simulink model "Filter_attivo"  (R2016b)
settings: Solver=ode23t  StartTime=0.0  StopTime=2.4  MaxStep=1e-4  RelTol=1e-3  EnableMultiTasking=on
values from neighbouring files (symbols this model uses):
  ampiezza_rete = 150/sqrt(3)    [Data.m]    (also in taratura.m)
  C = 2.2e-3    (= 0.0022)    [Data.m]
  C_raddr = 600e-6    (= 0.0006)    [Data.m]
  f = 50    [Data.m]    (also in Spettro_complesso.m = bar(-fp((26:25:25000-25)),PyTHD(length(PyTHD)-1:-1:length(Py)
  f_am = 500    [Data.m]
  h = Lagrange_coef(f,1/Tc)    [Data.m]    (also in Lagrange_coef.m = NaN(4,round(fc/f1*0.5)))
  h_rit = Lagrange_coef_rit(1.5)    [Data.m]
  k_interno = 0.99    [tuning.m]
  k_par_AM = 10    [Data.m]
  ki_PI = 0.2    [Data.m]
  ki_PLL = 1000    [Data.m]
  ki_ris = 47.5*2    (= 95)    [Data.m]
  kp_PI = 1.57    [Data.m]
  kp_PLL = 0.9    [Data.m]
  kp_ris = 47.5*0.089*2    (= 8.455)    [Data.m]
  L_disaccoppiamento = 2*1.18e-3    (= 0.00236)    [Data.m]    (also in taratura.m)
  L_rete = 4e-3    (= 0.004)    [Data.m]    (also in tuning.m)
  max_PI = 8    [Data.m]
  max_PLL = 1000    [Data.m]
  min_PI = -8    [Data.m]
  min_PLL = -1000    [Data.m]
  Notch_z = 1-Peaking_z    [Data.m]
  Notch_z_AM1 = 1-Peaking_z_AM1    [Notch.m]
  peak_rete = Peaking(f,1/Tc,0.1)    [Data.m]
  Peaking_dir1_d = c2d(Peaking_dir1_s,1/fs,'tustin')    [semipeaking.m]
  pendenza = 1000    [Data.m]
  R_carico = 50    [Data.m]
  R_disaccoppiamento = 2*13e-3    (= 0.026)    [Data.m]    (also in taratura.m)
  R_raddr = 60    [Data.m]
  R_rete = 100e-3    (= 0.1)    [Data.m]    (also in tuning.m = 0.01)
  T = 20e-3    (= 0.02)    [Data.m]    (also in tuning.m)
  tau_filtro_Vdc_ref = 0.15    [Data.m]
  Tc = 1/10000    (= 0.0001)    [Data.m]    (also in taratura.m; tuning.m)
  Vdc_ref = 200    [Data.m]    (also in taratura.m)
  w_filtro = 2*pi*f_taglio    (= 56548.6677646)    [Data.m]
undefined symbols (not defined in the file or in its folder): DiscIntNeverNeededParam, k_par, k_ser, Notch_z_AM1_5, Notch_z_AM1_7, Notch_z_AM2_5, Notch_z_AM2_7, Peaking_inv_d, plecs, Q_inv
libraries: powerlib x54, simulink x8, powerlib_extras x4, powerlib_meascontrol x2
(part 2 of 5)

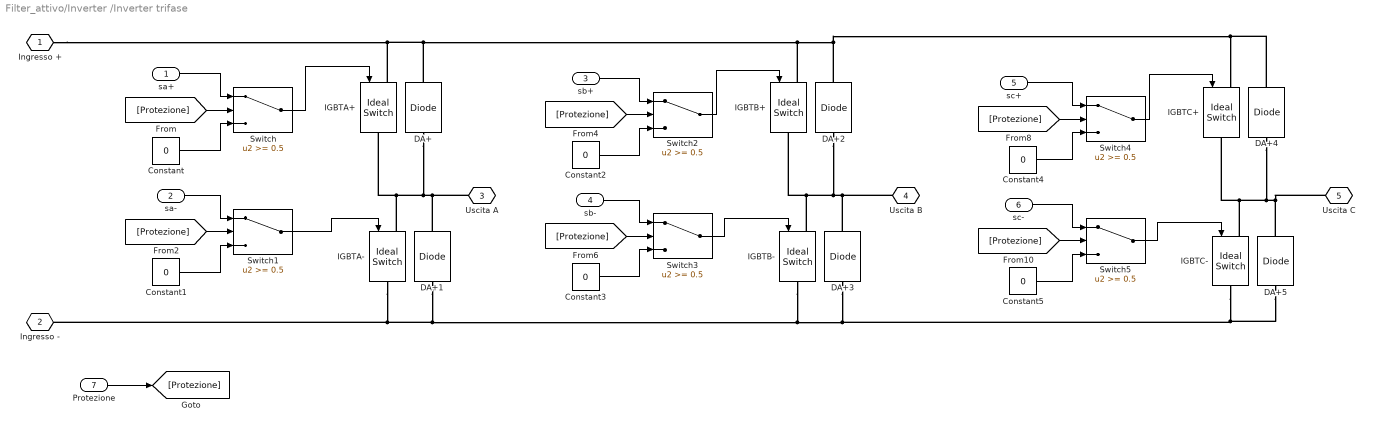
== system Filter_attivo/Inverter /Inverter trifase ==
  sa+ : Inport
  sa- : Inport  Port=2
  sb+ : Inport  Port=3
  sb- : Inport  Port=4
  sc+ : Inport  Port=5
  sc- : Inport  Port=6
  Protezione : Inport  Port=7
  Constant{,1..5} (6 alike) : Constant  Value=0
  DA+{,1..5} (6 alike) : powerlib/Power Electronics/Diode  Ron=Resistance_D  Lon=0  Vf=Forw_volt_d  IC=0  UseSnubber=off  Rs=500  Cs=250e-9  Measurements=off
  IGBTA+ : powerlib/Power Electronics/Ideal Switch  Ron=Int_res  Lon=0  IC=0  Rs=Snubber_res  Cs=inf  Measurements=off
  IGBTA- : powerlib/Power Electronics/Ideal Switch  Ron=Int_res  Lon=0  IC=0  Rs=Snubber_res  Cs=inf  Measurements=off
  IGBTB+ : powerlib/Power Electronics/Ideal Switch  Ron=Int_res  Lon=0  IC=0  Rs=Snubber_res  Cs=inf  Measurements=off
  IGBTB- : powerlib/Power Electronics/Ideal Switch  Ron=Int_res  Lon=0  IC=0  Rs=Snubber_res  Cs=inf  Measurements=off
  IGBTC+ : powerlib/Power Electronics/Ideal Switch  Ron=Int_res  Lon=0  IC=0  Rs=Snubber_res  Cs=inf  Measurements=off
  IGBTC- : powerlib/Power Electronics/Ideal Switch  Ron=Int_res  Lon=0  IC=0  Rs=Snubber_res  Cs=inf  Measurements=off
  Switch{,1..5} (6 alike) : Switch  Threshold=0.5
  Ingresso + : PMIOPort  Tag=PMCPort  Port=1  Side=Left
  Ingresso - : PMIOPort  Tag=PMCPort  Port=2  Side=Left
  Uscita A : PMIOPort  Tag=PMCPort  Port=3  Side=Right
  Uscita B : PMIOPort  Tag=PMCPort  Port=4  Side=Right
  Uscita C : PMIOPort  Tag=PMCPort  Port=5  Side=Right
  wires:
  Switch/1 -> IGBTA+/1
  [Protezione] -> Switch/2
  sa+/1 -> Switch/1
  sa-/1 -> Switch1/1
  [Protezione] -> Switch1/2
  [Protezione] -> Switch2/2
  sb+/1 -> Switch2/1
  sb-/1 -> Switch3/1
  [Protezione] -> Switch3/2
  [Protezione] -> Switch4/2
  sc+/1 -> Switch4/1
  sc-/1 -> Switch5/1
  [Protezione] -> Switch5/2
  Constant/1 -> Switch/3
  Constant1/1 -> Switch1/3
  Constant2/1 -> Switch2/3
  Constant3/1 -> Switch3/3
  Constant4/1 -> Switch4/3
  Constant5/1 -> Switch5/3
  Protezione/1 -> [Protezione]
  Switch1/1 -> IGBTA-/1
  Switch3/1 -> IGBTB-/1
  Switch2/1 -> IGBTB+/1
  Switch5/1 -> IGBTC-/1
  Switch4/1 -> IGBTC+/1
  connections:
  DA+1/LConn1 -- IGBTA-/RConn1 -- Ingresso -/RConn1 -- IGBTB-/RConn1 -- DA+5/LConn1 -- IGBTC-/RConn1 -- DA+3/LConn1
  DA+/LConn1 -- DA+1/RConn1 -- Uscita A/RConn1 -- IGBTA-/LConn1 -- IGBTA+/RConn1
  IGBTA+/LConn1 -- Ingresso +/RConn1 -- DA+/RConn1 -- IGBTB+/LConn1 -- DA+4/RConn1 -- IGBTC+/LConn1 -- DA+2/RConn1
  IGBTB+/RConn1 -- IGBTB-/LConn1 -- Uscita B/RConn1 -- DA+3/RConn1 -- DA+2/LConn1
  IGBTC+/RConn1 -- IGBTC-/LConn1 -- Uscita C/RConn1 -- DA+5/RConn1 -- DA+4/LConn1

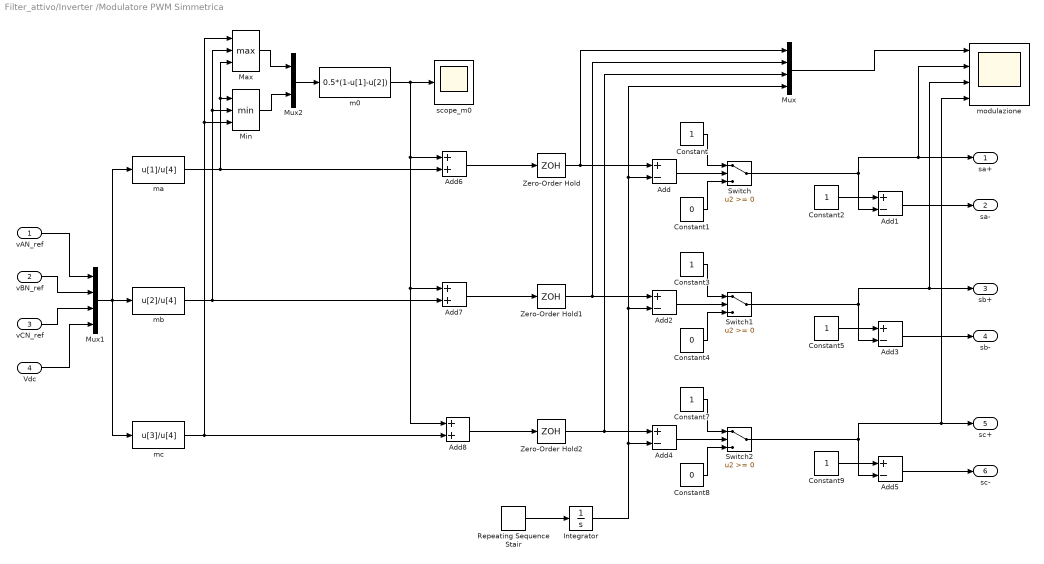
== system Filter_attivo/Inverter /Modulatore PWM Simmetrica ==
  vAN_ref : Inport
  vBN_ref : Inport  Port=2
  vCN_ref : Inport  Port=3
  Vdc : Inport  Port=4
  Add{,1..5} (6 alike) : Sum  Inputs=+-
  Add6 : Sum
  Add7 : Sum
  Add8 : Sum
  Constant{,2..3,5,7,9} (6 alike) : Constant
  Constant1 : Constant  Value=0
  Constant4 : Constant  Value=0
  Constant8 : Constant  Value=0
  Integrator : Integrator
  Max : MinMax  Function=max  Inputs=3
  Min : MinMax  Inputs=3
  Mux : Mux
  Mux1 : Mux
  Mux2 : Mux  Inputs=2
  Repeating Sequence Stair : simulink/Sources/Repeating Sequence Stair  OutValues=[2/Tc -2/Tc].'  tsamp=Tc/2  OutMin=[]  OutMax=[]  OutDataTypeStr=float('double')  OutputDataTypeScalingMode=Specify via dialog  OutDataType=float('double')  ConRadixGroup=Best Precision: Vector-wise  OutScaling=2^-12
  Switch : Switch
  Switch1 : Switch
  Switch2 : Switch
  Zero-Order Hold : ZeroOrderHold  SampleTime=Tc
  Zero-Order Hold1 : ZeroOrderHold  SampleTime=Tc
  Zero-Order Hold2 : ZeroOrderHold  SampleTime=Tc
  m0 : Fcn  Expr=0.5*(1-u[1]-u[2])
  ma : Fcn  Expr=u[1]/u[4]
  mb : Fcn  Expr=u[2]/u[4]
  mc : Fcn  Expr=u[3]/u[4]
  modulazione : Scope  NumInputPorts=4
  scope_m0 : Scope
  sa+ : Outport
  sa- : Outport  Port=2
  sb+ : Outport  Port=3
  sb- : Outport  Port=4
  sc+ : Outport  Port=5
  sc- : Outport  Port=6
  wires:
  Zero-Order Hold/1 -> Add/1, Mux/1
  Integrator/1 -> Add2/2, Add/2, Mux/4, Add4/2
  Add/1 -> Switch/2
  Constant/1 -> Switch/1
  Constant1/1 -> Switch/3
  Switch/1 -> Add1/2, sa+/1, modulazione/2
  Constant2/1 -> Add1/1
  Add1/1 -> sa-/1
  Repeating Sequence Stair/1 -> Integrator/1
  Zero-Order Hold1/1 -> Add2/1, Mux/2
  Add2/1 -> Switch1/2
  Constant3/1 -> Switch1/1
  Constant4/1 -> Switch1/3
  Switch1/1 -> Add3/2, sb+/1, modulazione/3
  Constant5/1 -> Add3/1
  Add3/1 -> sb-/1
  vAN_ref/1 -> Mux1/1
  vBN_ref/1 -> Mux1/2
  vCN_ref/1 -> Mux1/3
  Vdc/1 -> Mux1/4
  Zero-Order Hold2/1 -> Add4/1, Mux/3
  Add4/1 -> Switch2/2
  Constant7/1 -> Switch2/1
  Constant8/1 -> Switch2/3
  Switch2/1 -> Add5/2, sc+/1, modulazione/4
  Constant9/1 -> Add5/1
  Add5/1 -> sc-/1
  Mux1/1 -> ma/1, mc/1, mb/1
  Mux/1 -> modulazione/1
  mb/1 -> Min/2, Max/2, Add7/2
  mc/1 -> Min/3, Max/1, Add8/2
  ma/1 -> Min/1, Max/3, Add6/2
  Min/1 -> Mux2/2
  Max/1 -> Mux2/1
  Add6/1 -> Zero-Order Hold/1
  Add8/1 -> Zero-Order Hold2/1
  Add7/1 -> Zero-Order Hold1/1
  m0/1 -> scope_m0/1, Add6/1, Add7/1, Add8/1
  Mux2/1 -> m0/1

== system Filter_attivo/Inverter /Scope_idc ==
  1 : Inport
  " InputMux " : Subsystem
      mask Display: disp('Mux')
  " S-Function " : S-Function  FunctionName=plecs  SFunctionDeploymentMode=off  EnableBusSupport=off
  wires:
  " InputMux "/1(Out) -> " S-Function "/1
  1/1 -> " InputMux "/1(In1)

== system Filter_attivo/Inverter /Scope_idc_media ==
  1 : Inport
  " InputMux " : Subsystem
      mask Display: disp('Mux')
  " S-Function " : S-Function  FunctionName=plecs  SFunctionDeploymentMode=off  EnableBusSupport=off
  wires:
  1/1 -> " InputMux "/1(In1)
  " InputMux "/1(Out) -> " S-Function "/1

== system Filter_attivo/Protezione/Scope ==
  1 : Inport
  2 : Inport  Port=2
  3 : Inport  Port=3
  " 1 " : DataTypeConversion  SaturateOnIntegerOverflow=on  RndMeth=Zero
  " 2 " : DataTypeConversion  SaturateOnIntegerOverflow=on  RndMeth=Zero
  " 3 " : DataTypeConversion  SaturateOnIntegerOverflow=on  RndMeth=Zero
  " InputMux " : Mux  Inputs=3
  " S-Function " : S-Function  FunctionName=plecs  SFunctionDeploymentMode=off  EnableBusSupport=off
  wires:
  " InputMux "/1 -> " S-Function "/1
  1/1 -> " 1 "/1
  " 1 "/1 -> " InputMux "/1
  2/1 -> " 2 "/1
  " 2 "/1 -> " InputMux "/2
  3/1 -> " 3 "/1
  " 3 "/1 -> " InputMux "/3

== system Filter_attivo/Rete/D ==
  ab(c) : Inport
  Gain : Gain  Gain=[1 0; 1/sqrt(3) 2/sqrt(3)]  Multiplication=Matrix(K*u)
  dq(0) : Outport
  wires:
  Gain/1 -> dq(0)/1
  ab(c)/1 -> Gain/1

== system Filter_attivo/Rete/Integratore discreto con reset a 2*pi ==
  omega : Inport
  Add : Sum
  Compare To Zero : simulink/Logic and Bit Operations/Compare To Zero  relop=>  OutDataTypeStr=uint8  ZeroCross=off
  Constant : Constant  Value=2*pi
  Constant1 : Constant  Value=-2*pi
  Constant2 : Constant  Value=-2*pi
  Constant3 : Constant  Value=2*pi
  Discrete-Time Integrator : DiscreteIntegrator  ExternalReset=rising  InitialConditionSource=external  SampleTime=Tc  ShowStatePort=on  ICPrevOutput=DiscIntNeverNeededParam  ICPrevScaledInput=DiscIntNeverNeededParam
  Logical Operator2 : Logic  Operator=OR  AllPortsSameDT=off  OutDataTypeStr=boolean
  Relational Operator : RelationalOperator  Operator=<=  OutDataTypeStr=boolean  RndMeth=Nearest
  Relational Operator1 : RelationalOperator  Operator=<=  OutDataTypeStr=boolean  RndMeth=Nearest
  Switch : Switch  Threshold=0.5
  teta : Outport
  wires:
  Logical Operator2/1 -> Discrete-Time Integrator/2
  Relational Operator/1 -> Logical Operator2/1
  Relational Operator1/1 -> Logical Operator2/2
  Discrete-Time Integrator/State -> Add/1, Compare To Zero/1, Relational Operator1/1, Relational Operator/2
  Constant/1 -> Relational Operator/1
  Constant1/1 -> Relational Operator1/2
  omega/1 -> Discrete-Time Integrator/1
  Discrete-Time Integrator/1 -> teta/1
  Constant2/1 -> Switch/1
  Constant3/1 -> Switch/3
  Switch/1 -> Add/2
  Compare To Zero/1 -> Switch/2
  Add/1 -> Discrete-Time Integrator/3

== system Filter_attivo/Rete/generatore diretta e inversa ==
  note: c'è un disagio forte, perchè tutto il sistema è sincronizzato con una inversa e non con una diretta.
  Frequenza1 : Constant  Value=fase_i
  Frequenza2 : Constant  Value=f
  Gain1 : Gain  Gain=2*pi
  Gain2 : Gain  Gain=ampiezza_i
  Gain3 : Gain  Gain=pi/180
  MATLAB Function : MATLAB Function  TreatAsAtomicUnit=on
  Mux : Mux  Inputs=3
  Ramp2 : simulink/Sources/Ramp  slope=pendenza  start=0  X0=0
  Scope1 : Subsystem  LoadFcn=plecs('sl', 300);  InitFcn=plecs('sl', 314);  StartFcn=plecs('sl', 308);  StopFcn=plecs('sl', 309);  mask{Settings=<binary blob, 876 chars, not shown>}
      mask init:
      | plecs('sl', 315);
      settings: CopyFcn=plecs('sl', 303);  DeleteFcn=plecs('sl', 305);  UndoDeleteFcn=plecs('sl', 306);  PreSaveFcn=plecs('sl', 311);  NameChangeFcn=plecs('sl', 310);  DestroyFcn=plecs('sl', 307);  OpenFcn=plecs('sl', 302);  ErrorFcn=plerrorfcn
      mask Display: plot([0.1 0.9 0.9 0.1 0.1], [0.9 0.9 0.5 0.5 0.9])
  Step3 : Step  Time=0  After=ampiezza_rete  SampleTime=0
  Switch3 : Switch  Threshold=ampiezza_rete
  "integratore con reset " : Subsystem
  v_a : Outport
  v_b : Outport  Port=2
  v_c : Outport  Port=3
  wires:
  Gain1/1 -> "integratore con reset "/1(omega)
  Ramp2/1 -> Switch3/2, Switch3/3
  Step3/1 -> Switch3/1
  Frequenza2/1 -> Gain1/1
  "integratore con reset "/1(teta) -> MATLAB Function/1(teta)
  Switch3/1 -> Gain2/1, MATLAB Function/2(a_d)
  MATLAB Function/1(v_a) -> Mux/1, v_a/1
  MATLAB Function/3(v_c) -> Mux/3, v_b/1
  MATLAB Function/2(v_b) -> Mux/2, v_c/1
  Gain2/1 -> MATLAB Function/3(a_i)
  Frequenza1/1 -> Gain3/1
  Mux/1 -> Scope1/1(1)
  Gain3/1 -> MATLAB Function/4(fase_i)

== system Filter_attivo/Scope1/ InputMux  ==
  In1 : Inport
  Convert1 : DataTypeConversion  SaturateOnIntegerOverflow=on  RndMeth=Zero
  Mux : Mux  Inputs=1
  Out : Outport
  wires:
  Convert1/1 -> Mux/1
  In1/1 -> Convert1/1
  Mux/1 -> Out/1

== system Filter_attivo/Scope2/ InputMux  ==
  In1 : Inport
  Convert1 : DataTypeConversion  SaturateOnIntegerOverflow=on  RndMeth=Zero
  Mux : Mux  Inputs=1
  Out : Outport
  wires:
  Mux/1 -> Out/1
  In1/1 -> Convert1/1
  Convert1/1 -> Mux/1

== system Filter_attivo/Tensione bus DC/ InputMux  ==
  In1 : Inport
  Convert1 : DataTypeConversion  SaturateOnIntegerOverflow=on  RndMeth=Zero
  Mux : Mux  Inputs=1
  Out : Outport
  wires:
  Convert1/1 -> Mux/1
  In1/1 -> Convert1/1
  Mux/1 -> Out/1

== system Filter_attivo/XY Plot/ InputMux  ==
  In1 : Inport
  In2 : Inport  Port=2
  Convert1 : DataTypeConversion  SaturateOnIntegerOverflow=on  RndMeth=Zero
  Convert2 : DataTypeConversion  SaturateOnIntegerOverflow=on  RndMeth=Zero
  Mux : Mux  Inputs=2
  Out : Outport
  wires:
  Convert2/1 -> Mux/2
  In2/1 -> Convert2/1
  Convert1/1 -> Mux/1
  In1/1 -> Convert1/1
  Mux/1 -> Out/1

== system Filter_attivo/v_rete/ InputMux  ==
  In1 : Inport
  Convert1 : DataTypeConversion  SaturateOnIntegerOverflow=on  RndMeth=Zero
  Mux : Mux  Inputs=1
  Out : Outport
  wires:
  Mux/1 -> Out/1
  In1/1 -> Convert1/1
  Convert1/1 -> Mux/1

== system Filter_attivo/v_rete1/ InputMux  ==
  In1 : Inport
  Convert1 : DataTypeConversion  SaturateOnIntegerOverflow=on  RndMeth=Zero
  Mux : Mux  Inputs=1
  Out : Outport
  wires:
  Convert1/1 -> Mux/1
  In1/1 -> Convert1/1
  Mux/1 -> Out/1

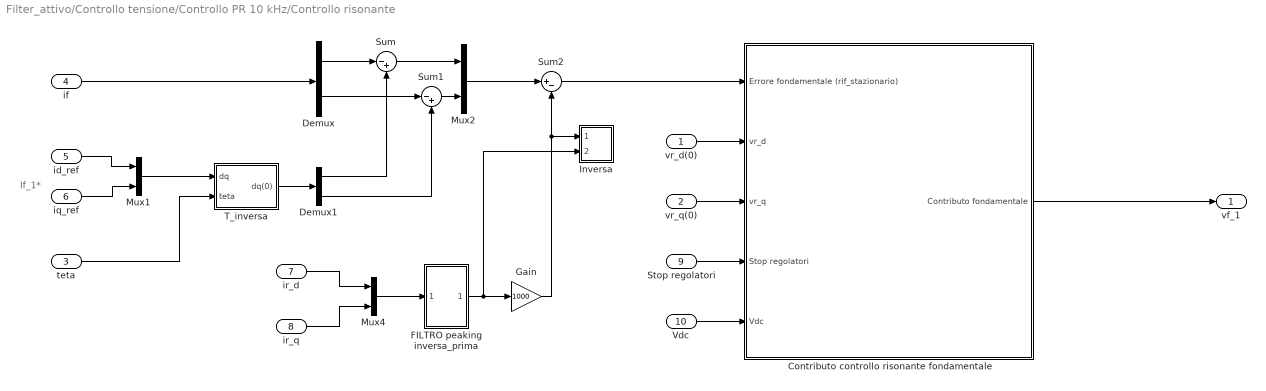
== system Filter_attivo/Controllo tensione/Controllo PR 10 kHz/Controllo risonante ==
  note: If_1*
  vr_d(0) : Inport
  vr_q(0) : Inport  Port=2
  teta : Inport  Port=3
  if : Inport  Port=4
  id_ref : Inport  Port=5
  iq_ref : Inport  Port=6
  ir_d : Inport  Port=7
  ir_q : Inport  Port=8
  Stop regolatori : Inport  Port=9
  Vdc : Inport  Port=10
  Contributo controllo risonante fondamentale : Subsystem
  Demux : Demux  Outputs=2
  Demux1 : Demux  Outputs=2
  FILTRO peaking inversa_prima : Subsystem
  Gain : Gain  Gain=1000
  Inversa : Subsystem  LoadFcn=plecs('sl', 300);  InitFcn=plecs('sl', 314);  StartFcn=plecs('sl', 308);  StopFcn=plecs('sl', 309);  mask{Settings=<binary blob, 1020 chars, not shown>}
      mask init:
      | plecs('sl', 315);
      settings: CopyFcn=plecs('sl', 303);  DeleteFcn=plecs('sl', 305);  UndoDeleteFcn=plecs('sl', 306);  PreSaveFcn=plecs('sl', 311);  NameChangeFcn=plecs('sl', 310);  DestroyFcn=plecs('sl', 307);  OpenFcn=plecs('sl', 302);  ErrorFcn=plerrorfcn
      mask Display: plot([0.1 0.9 0.9 0.1 0.1], [0.9 0.9 0.5 0.5 0.9])
  Mux1 : Mux  Inputs=2
  Mux2 : Mux  Inputs=2
  Mux4 : Mux  Inputs=2
  Sum : Sum  Inputs=|-+
  Sum1 : Sum  Inputs=|-+
  Sum2 : Sum  Inputs=|+-
  T_inversa : Subsystem
  vf_1 : Outport
  wires:
  Demux/1 -> Sum/1
  Demux/2 -> Sum1/1
  id_ref/1 -> Mux1/1
  iq_ref/1 -> Mux1/2
  Demux1/1 -> Sum/2
  Demux1/2 -> Sum1/2
  Sum/1 -> Mux2/1
  Sum1/1 -> Mux2/2
  vr_d(0)/1 -> Contributo controllo risonante fondamentale/2(vr_d)
  vr_q(0)/1 -> Contributo controllo risonante fondamentale/3(vr_q)
  Contributo controllo risonante fondamentale/1("Contributo fondamentale ") -> vf_1/1
  Mux2/1 -> Sum2/1
  teta/1 -> T_inversa/2(teta)
  Mux1/1 -> T_inversa/1(dq)
  T_inversa/1(dq(0)) -> Demux1/1
  Stop regolatori/1 -> Contributo controllo risonante fondamentale/4(Stop regolatori)
  Mux4/1 -> FILTRO peaking inversa_prima/1(In2)
  ir_d/1 -> Mux4/1
  ir_q/1 -> Mux4/2
  FILTRO peaking inversa_prima/1(Out1) -> Gain/1, Inversa/2(2)
  Gain/1 -> Sum2/2, Inversa/1(1)
  Sum2/1 -> Contributo controllo risonante fondamentale/1(Errore fondamentale (rif_stazionario))
  Vdc/1 -> Contributo controllo risonante fondamentale/5(Vdc)
  if/1 -> Demux/1

== system Filter_attivo/Controllo tensione/Controllo PR 10 kHz/D ==
  ab(c) : Inport
  Gain : Gain  Gain=[1 0; 1/sqrt(3) 2/sqrt(3)]  Multiplication=Matrix(K*u)
  dq(0) : Outport
  wires:
  Gain/1 -> dq(0)/1
  ab(c)/1 -> Gain/1

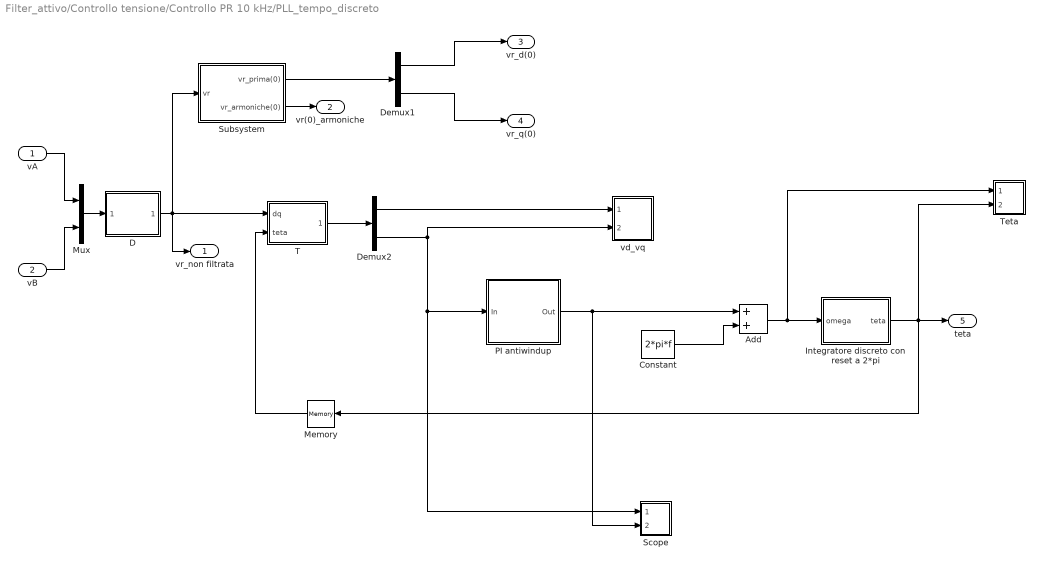
== system Filter_attivo/Controllo tensione/Controllo PR 10 kHz/PLL_tempo_discreto ==
  vA : Inport
  vB : Inport  Port=2
  Add : Sum
  Constant : Constant  Value=2*pi*f
  D : Subsystem
  Demux1 : Demux  Outputs=2
  Demux2 : Demux  Outputs=2
  Integratore discreto con reset a 2*pi : Subsystem
  Memory : Memory  InheritSampleTime=on
  Mux : Mux  Inputs=2
  PI antiwindup : Subsystem  mask{kp_PLL_edit=0.5, ki_PLL_edit=500}
      mask prompts: kp_PLL_edit "kp"; ki_PLL_edit "ki"
  Scope : Subsystem  LoadFcn=plecs('sl', 300);  InitFcn=plecs('sl', 314);  StartFcn=plecs('sl', 308);  StopFcn=plecs('sl', 309);  mask{Settings=<binary blob, 1004 chars, not shown>}
      mask init:
      | plecs('sl', 315);
      settings: CopyFcn=plecs('sl', 303);  DeleteFcn=plecs('sl', 305);  UndoDeleteFcn=plecs('sl', 306);  PreSaveFcn=plecs('sl', 311);  NameChangeFcn=plecs('sl', 310);  DestroyFcn=plecs('sl', 307);  OpenFcn=plecs('sl', 302);  ErrorFcn=plerrorfcn
      mask Display: plot([0.1 0.9 0.9 0.1 0.1], [0.9 0.9 0.5 0.5 0.9])
  Subsystem : Subsystem
  T : Subsystem
  Teta : Subsystem  LoadFcn=plecs('sl', 300);  InitFcn=plecs('sl', 314);  StartFcn=plecs('sl', 308);  StopFcn=plecs('sl', 309);  mask{Settings=<binary blob, 1020 chars, not shown>}
      mask init:
      | plecs('sl', 315);
      settings: CopyFcn=plecs('sl', 303);  DeleteFcn=plecs('sl', 305);  UndoDeleteFcn=plecs('sl', 306);  PreSaveFcn=plecs('sl', 311);  NameChangeFcn=plecs('sl', 310);  DestroyFcn=plecs('sl', 307);  OpenFcn=plecs('sl', 302);  ErrorFcn=plerrorfcn
      mask Display: plot([0.1 0.9 0.9 0.1 0.1], [0.9 0.9 0.5 0.5 0.9])
  vd_vq : Subsystem  LoadFcn=plecs('sl', 300);  InitFcn=plecs('sl', 314);  StartFcn=plecs('sl', 308);  StopFcn=plecs('sl', 309);  mask{Settings=<binary blob, 300 chars, not shown>}
      mask init:
      | plecs('sl', 315);
      settings: CopyFcn=plecs('sl', 303);  DeleteFcn=plecs('sl', 305);  UndoDeleteFcn=plecs('sl', 306);  PreSaveFcn=plecs('sl', 311);  NameChangeFcn=plecs('sl', 310);  DestroyFcn=plecs('sl', 307);  OpenFcn=plecs('sl', 302);  ErrorFcn=plerrorfcn
      mask Display: plot([0.1 0.9 0.9 0.1 0.1], [0.9 0.9 0.5 0.5 0.9])
  vr_non filtrata : Outport
  vr(0)_armoniche : Outport  Port=2
  vr_d(0) : Outport  Port=3
  vr_q(0) : Outport  Port=4
  teta : Outport  Port=5
  wires:
  Add/1 -> Teta/1(1), Integratore discreto con reset a 2*pi/1(omega)
  Constant/1 -> Add/2
  T/1(dq(teta)) -> Demux2/1
  Demux2/1 -> vd_vq/1(1)
  Integratore discreto con reset a 2*pi/1(teta) -> Memory/1, teta/1, Teta/2(2)
  Memory/1 -> T/2(teta)
  PI antiwindup/1(Out) -> Scope/2(2), Add/1
  vA/1 -> Mux/1
  vB/1 -> Mux/2
  Mux/1 -> D/1(ab(c))
  D/1(dq(0)) -> vr_non filtrata/1, Subsystem/1(vr), T/1(dq)
  Subsystem/2(vr_armoniche(0)) -> vr(0)_armoniche/1
  Demux1/1 -> vr_d(0)/1
  Demux1/2 -> vr_q(0)/1
  Subsystem/1(vr_prima(0)) -> Demux1/1
  Demux2/2 -> vd_vq/2(2), PI antiwindup/1(In), Scope/1(1)

== system Filter_attivo/Controllo tensione/Controllo PR 10 kHz/Scope ==
  1 : Inport
  " InputMux " : Subsystem
      mask Display: disp('Mux')
  " S-Function " : S-Function  FunctionName=plecs  SFunctionDeploymentMode=off  EnableBusSupport=off
  wires:
  1/1 -> " InputMux "/1(In1)
  " InputMux "/1(Out) -> " S-Function "/1

== system Filter_attivo/Controllo tensione/Controllo PR 10 kHz/Scope2 ==
  1 : Inport
  2 : Inport  Port=2
  " 1 " : DataTypeConversion  SaturateOnIntegerOverflow=on  RndMeth=Zero
  " 2 " : DataTypeConversion  SaturateOnIntegerOverflow=on  RndMeth=Zero
  " InputMux " : Mux  Inputs=2
  " S-Function " : S-Function  FunctionName=plecs  SFunctionDeploymentMode=off  EnableBusSupport=off
  wires:
  " InputMux "/1 -> " S-Function "/1
  1/1 -> " 1 "/1
  " 1 "/1 -> " InputMux "/1
  2/1 -> " 2 "/1
  " 2 "/1 -> " InputMux "/2

== system Filter_attivo/Controllo tensione/Controllo PR 10 kHz/controllo  ==
  teta : Inport
  ir : Inport  Port=2
  Demux : Demux  Outputs=2
  Mux : Mux  Inputs=2
  PI antiwindup : Subsystem  mask{kp_rifasamento=0.05, ki_rifasamento=5}
      mask prompts: kp_rifasamento "kp"; ki_rifasamento "ki"
  Peaking 1^ armonica : DiscreteTransferFcn  Numerator=cell2mat(peak_rete.num)  Denominator=cell2mat(peak_rete.den)
  Scope : Subsystem  LoadFcn=plecs('sl', 300);  InitFcn=plecs('sl', 314);  StartFcn=plecs('sl', 308);  StopFcn=plecs('sl', 309);  mask{Settings=<binary blob, 892 chars, not shown>}
      mask init:
      | plecs('sl', 315);
      settings: CopyFcn=plecs('sl', 303);  DeleteFcn=plecs('sl', 305);  UndoDeleteFcn=plecs('sl', 306);  PreSaveFcn=plecs('sl', 311);  NameChangeFcn=plecs('sl', 310);  DestroyFcn=plecs('sl', 307);  OpenFcn=plecs('sl', 302);  ErrorFcn=plerrorfcn
      mask Display: plot([0.1 0.9 0.9 0.1 0.1], [0.9 0.9 0.5 0.5 0.9])
  Scope1 : Subsystem  LoadFcn=plecs('sl', 300);  InitFcn=plecs('sl', 314);  StartFcn=plecs('sl', 308);  StopFcn=plecs('sl', 309);  mask{Settings=<binary blob, 892 chars, not shown>}
      mask init:
      | plecs('sl', 315);
      settings: CopyFcn=plecs('sl', 303);  DeleteFcn=plecs('sl', 305);  UndoDeleteFcn=plecs('sl', 306);  PreSaveFcn=plecs('sl', 311);  NameChangeFcn=plecs('sl', 310);  DestroyFcn=plecs('sl', 307);  OpenFcn=plecs('sl', 302);  ErrorFcn=plerrorfcn
      mask Display: plot([0.1 0.9 0.9 0.1 0.1], [0.9 0.9 0.5 0.5 0.9])
  Scope2 : Subsystem  LoadFcn=plecs('sl', 300);  InitFcn=plecs('sl', 314);  StartFcn=plecs('sl', 308);  StopFcn=plecs('sl', 309);  mask{Settings=<binary blob, 892 chars, not shown>}
      mask init:
      | plecs('sl', 315);
      settings: CopyFcn=plecs('sl', 303);  DeleteFcn=plecs('sl', 305);  UndoDeleteFcn=plecs('sl', 306);  PreSaveFcn=plecs('sl', 311);  NameChangeFcn=plecs('sl', 310);  DestroyFcn=plecs('sl', 307);  OpenFcn=plecs('sl', 302);  ErrorFcn=plerrorfcn
      mask Display: plot([0.1 0.9 0.9 0.1 0.1], [0.9 0.9 0.5 0.5 0.9])
  Scope3 : Subsystem  LoadFcn=plecs('sl', 300);  InitFcn=plecs('sl', 314);  StartFcn=plecs('sl', 308);  StopFcn=plecs('sl', 309);  mask{Settings=<binary blob, 892 chars, not shown>}
      mask init:
      | plecs('sl', 315);
      settings: CopyFcn=plecs('sl', 303);  DeleteFcn=plecs('sl', 305);  UndoDeleteFcn=plecs('sl', 306);  PreSaveFcn=plecs('sl', 311);  NameChangeFcn=plecs('sl', 310);  DestroyFcn=plecs('sl', 307);  OpenFcn=plecs('sl', 302);  ErrorFcn=plerrorfcn
      mask Display: plot([0.1 0.9 0.9 0.1 0.1], [0.9 0.9 0.5 0.5 0.9])
  Scope6 : Scope
  Step1 : Step  Time=avvio_rifasamento
  Sum5 : Sum  Inputs=|-+
  Switch : Switch  Criteria=u2 > Threshold
  T : Subsystem
  ir_q : Constant  Value=0
  ir_q1 : Constant  Value=0
  if_q* : Outport
  wires:
  Mux/1 -> Scope/1(1)
  ir/1 -> Peaking 1^ armonica/1
  T/1(dq(teta)) -> Scope1/1(1), Demux/1
  Sum5/1 -> PI antiwindup/1(In)
  Peaking 1^ armonica/1 -> Scope2/1(1), T/1(dq)
  Demux/2 -> Mux/2, Switch/1
  teta/1 -> T/2(teta)
  PI antiwindup/1(Out) -> Scope6/1, Scope3/1(1), if_q*/1
  ir_q/1 -> Mux/1, Sum5/2
  Switch/1 -> Sum5/1
  Step1/1 -> Switch/2
  ir_q1/1 -> Switch/3

== system Filter_attivo/Controllo tensione/Controllo PR 10 kHz/controllo bus DC ==
  Vdc : Inport
  Avvio Inverter : Inport  Port=2
  Filtro passa-basso tempo discreto : Subsystem
  PI antiwindup : Subsystem
  PI antiwindup1 : Subsystem  mask{kp_rifasamento=0.3, ki_rifasamento=0.01}
      mask prompts: kp_rifasamento "kp"; ki_rifasamento "ki"
  Scope1 : Subsystem  LoadFcn=plecs('sl', 300);  InitFcn=plecs('sl', 314);  StartFcn=plecs('sl', 308);  StopFcn=plecs('sl', 309);  mask{Settings=<binary blob, 904 chars, not shown>}
      mask init:
      | plecs('sl', 315);
      settings: CopyFcn=plecs('sl', 303);  DeleteFcn=plecs('sl', 305);  UndoDeleteFcn=plecs('sl', 306);  PreSaveFcn=plecs('sl', 311);  NameChangeFcn=plecs('sl', 310);  DestroyFcn=plecs('sl', 307);  OpenFcn=plecs('sl', 302);  ErrorFcn=plerrorfcn
      mask Display: plot([0.1 0.9 0.9 0.1 0.1], [0.9 0.9 0.5 0.5 0.9])
  Scope2 : Subsystem  LoadFcn=plecs('sl', 300);  InitFcn=plecs('sl', 314);  StartFcn=plecs('sl', 308);  StopFcn=plecs('sl', 309);  mask{Settings=<binary blob, 1076 chars, not shown>}
      mask init:
      | plecs('sl', 315);
      settings: CopyFcn=plecs('sl', 303);  DeleteFcn=plecs('sl', 305);  UndoDeleteFcn=plecs('sl', 306);  PreSaveFcn=plecs('sl', 311);  NameChangeFcn=plecs('sl', 310);  DestroyFcn=plecs('sl', 307);  OpenFcn=plecs('sl', 302);  ErrorFcn=plerrorfcn
      mask Display: plot([0.1 0.9 0.9 0.1 0.1], [0.9 0.9 0.5 0.5 0.9])
  Scope6 : Scope
  Sum5 : Sum  Inputs=|+-
  Vdc_ref : Constant  Value=Vdc_ref
  id* : Outport
  wires:
  Filtro passa-basso tempo discreto/1(Vdc*_filtrata) -> Scope2/1(1), Sum5/1
  Vdc_ref/1 -> Filtro passa-basso tempo discreto/1(In)
  Sum5/1 -> PI antiwindup1/1(In)
  Vdc/1 -> Filtro passa-basso tempo discreto/3("Vdc "), Sum5/2
  Avvio Inverter/1 -> Filtro passa-basso tempo discreto/2(Avvio Inverter)
  PI antiwindup1/1(Out) -> Scope1/1(1), Scope6/1, id*/1

== system Filter_attivo/Controllo tensione/Controllo ripetitivo/Controllo ripetitivo ==
  Stop regolatori : Inport
  Avvio ripetitivo : Inport  Port=2
  "corrente rete " : Inport  Port=3
  teta : Inport  Port=4
  Trigger : TriggerPort  VariantControl=Variant
  Demux : Demux  Outputs=2
  Logical Operator1 : Logic  AllPortsSameDT=off  OutDataTypeStr=boolean
  Mux2 : Mux  Inputs=2
  Regolatore ripetitivo : Subsystem
  vf_h : Outport
  wires:
  Mux2/1 -> vf_h/1
  Demux/1 -> Regolatore ripetitivo/1(id*)
  Demux/2 -> Regolatore ripetitivo/2(iq*)
  "corrente rete "/1 -> Demux/1
  Regolatore ripetitivo/2(Out2) -> Mux2/2
  Regolatore ripetitivo/1(Out1) -> Mux2/1
  Avvio ripetitivo/1 -> Logical Operator1/1
  Logical Operator1/1 -> Regolatore ripetitivo/Enable
  Stop regolatori/1 -> Logical Operator1/2
  teta/1 -> Regolatore ripetitivo/3(teta)

== system Filter_attivo/Controllo tensione/Controllo ripetitivo/Controllo ripetitivo con downsampling ==
  Stop regolatori : Inport
  Avvio ripetitivo : Inport  Port=2
  "corrente rete " : Inport  Port=3
  Trigger : TriggerPort  VariantControl=Variant
  And : Logic  AllPortsSameDT=off  OutDataTypeStr=boolean
  Demux : Demux  Outputs=2
  Mux2 : Mux  Inputs=2
  Regolatore ripetitivo : Subsystem
  vf_h_DOWNSAMPLING : Outport
  wires:
  Stop regolatori/1 -> And/2
  And/1 -> Regolatore ripetitivo/Enable
  Avvio ripetitivo/1 -> And/1
  Regolatore ripetitivo/1(Out1) -> Mux2/1
  Regolatore ripetitivo/2(Out2) -> Mux2/2
  "corrente rete "/1 -> Demux/1
  Demux/2 -> Regolatore ripetitivo/2(iq*)
  Demux/1 -> Regolatore ripetitivo/1(id*)
  Mux2/1 -> vf_h_DOWNSAMPLING/1

== system Filter_attivo/Controllo tensione/Controllo ripetitivo/Notch Prima Armonica ==
  ir(a_b_c) : Inport
  Trigger : TriggerPort  VariantControl=Variant
  D : Subsystem
  Demux : Demux  Outputs=2
  "Filtro notch prima armonica " : Subsystem
  Filtro notch prima armonica 1 : Subsystem
  Gain : Gain  Gain=0.1
  Gain1 : Gain  Gain=0.9
  Mux : Mux  Inputs=2
  Sum : Sum  Inputs=|++
  ir_h(d_q) : Outport
  wires:
  Demux/2 -> Filtro notch prima armonica 1/1(ir)
  Demux/1 -> "Filtro notch prima armonica "/1(ir)
  D/1(dq(0)) -> Gain/1, Demux/1
  ir(a_b_c)/1 -> D/1(ab(c))
  "Filtro notch prima armonica "/1(irh) -> Mux/1
  Filtro notch prima armonica 1/1(irh) -> Mux/2
  Mux/1 -> Gain1/1
  Sum/1 -> ir_h(d_q)/1
  Gain/1 -> Sum/2
  Gain1/1 -> Sum/1

== system Filter_attivo/Controllo tensione/Scope/ InputMux  ==
  In1 : Inport
  Convert1 : DataTypeConversion  SaturateOnIntegerOverflow=on  RndMeth=Zero
  Mux : Mux  Inputs=1
  Out : Outport
  wires:
  Convert1/1 -> Mux/1
  In1/1 -> Convert1/1
  Mux/1 -> Out/1

== system Filter_attivo/Controllo tensione/Scope2/ InputMux  ==
  In1 : Inport
  Convert1 : DataTypeConversion  SaturateOnIntegerOverflow=on  RndMeth=Zero
  Mux : Mux  Inputs=1
  Out : Outport
  wires:
  Convert1/1 -> Mux/1
  In1/1 -> Convert1/1
  Mux/1 -> Out/1

== system Filter_attivo/Inverter /Scope_idc/ InputMux  ==
  In1 : Inport
  Convert1 : DataTypeConversion  SaturateOnIntegerOverflow=on  RndMeth=Zero
  Mux : Mux  Inputs=1
  Out : Outport
  wires:
  Mux/1 -> Out/1
  In1/1 -> Convert1/1
  Convert1/1 -> Mux/1

== system Filter_attivo/Inverter /Scope_idc_media/ InputMux  ==
  In1 : Inport
  Convert1 : DataTypeConversion  SaturateOnIntegerOverflow=on  RndMeth=Zero
  Mux : Mux  Inputs=1
  Out : Outport
  wires:
  Convert1/1 -> Mux/1
  In1/1 -> Convert1/1
  Mux/1 -> Out/1

== system Filter_attivo/Rete/generatore diretta e inversa/Scope1 ==
  1 : Inport
  " InputMux " : Subsystem
      mask Display: disp('Mux')
  " S-Function " : S-Function  FunctionName=plecs  SFunctionDeploymentMode=off  EnableBusSupport=off
  wires:
  " InputMux "/1(Out) -> " S-Function "/1
  1/1 -> " InputMux "/1(In1)

== system Filter_attivo/Rete/generatore diretta e inversa/integratore con reset  ==
  omega : Inport
  Add : Sum
  Compare To Zero : simulink/Logic and Bit Operations/Compare To Zero  relop=>  OutDataTypeStr=uint8  ZeroCross=off
  Constant : Constant  Value=2*pi
  Constant1 : Constant  Value=-2*pi
  Constant2 : Constant  Value=-2*pi
  Constant3 : Constant  Value=2*pi
  Integrator : Integrator  ExternalReset=rising  InitialConditionSource=external  ShowStatePort=on
  Logical Operator2 : Logic  Operator=OR  AllPortsSameDT=off  OutDataTypeStr=boolean
  Relational Operator : RelationalOperator  Operator=<=  OutDataTypeStr=boolean  RndMeth=Nearest
  Relational Operator1 : RelationalOperator  Operator=<=  OutDataTypeStr=boolean  RndMeth=Nearest
  Switch : Switch  Threshold=0.5
  teta : Outport
  wires:
  Logical Operator2/1 -> Integrator/2
  Relational Operator/1 -> Logical Operator2/1
  Relational Operator1/1 -> Logical Operator2/2
  Integrator/State -> Add/1, Compare To Zero/1, Relational Operator1/1, Relational Operator/2
  Constant/1 -> Relational Operator/1
  Constant1/1 -> Relational Operator1/2
  omega/1 -> Integrator/1
  Integrator/1 -> teta/1
  Constant2/1 -> Switch/1
  Constant3/1 -> Switch/3
  Switch/1 -> Add/2
  Compare To Zero/1 -> Switch/2
  Add/1 -> Integrator/3

== system Filter_attivo/Controllo tensione/Controllo PR 10 kHz/Controllo risonante/Contributo controllo risonante fondamentale ==
  note: vf1_q*
  note: vf1_d*
  Errore fondamentale (rif_stazionario) : Inport
  vr_d : Inport  Port=2
  vr_q : Inport  Port=3
  Stop regolatori : Inport  Port=4
  Vdc : Inport  Port=5
  Add : Sum  Inputs=-+
  Add1 : Sum  Inputs=+-
  Demux1 : Demux  Outputs=2
  Demux3 : Demux  Outputs=2
  Logical Operator : Logic  Operator=NOT  AllPortsSameDT=off  OutDataTypeStr=boolean
  Mux1 : Mux  Inputs=2
  Mux2 : Mux  Inputs=2
  PIR_tustin_prewarp : Subsystem  Commented=on  mask{w_ris=2*pi*f, kr_ris=ki_ris, kp_ris=kp_ris, Tc=Tc, delta=0}
      mask prompts: w_ris "frequenza risonanza"; kr_ris "guadagno risonante"; kp_ris "guadagno proporzionale"; Tc "Periodo di campionamento"; delta "attenuazione"
  PI_risonante : Subsystem
  "Contributo fondamentale " : Outport
  wires:
  Errore fondamentale (rif_stazionario)/1 -> Demux1/1
  Stop regolatori/1 -> Logical Operator/1
  vr_d/1 -> Add/2
  Demux3/2 -> Add1/2
  vr_q/1 -> Add1/1
  Mux2/1 -> Demux3/1
  Mux1/1 -> "Contributo fondamentale "/1
  Demux3/1 -> Add/1
  Vdc/1 -> PIR_tustin_prewarp/3(Vdc)
  Demux1/1 -> PI_risonante/1(In1)
  Demux1/2 -> PI_risonante/2(In2)
  PI_risonante/1(Out1) -> Mux2/1
  PI_risonante/2(Out2) -> Mux2/2
  Logical Operator/1 -> PI_risonante/Enable
  Add/1 -> Mux1/1
  Add1/1 -> Mux1/2

== system Filter_attivo/Controllo tensione/Controllo PR 10 kHz/Controllo risonante/FILTRO peaking inversa_prima ==
  In2 : Inport
  Demux : Demux  Outputs=2
  Discrete Transfer Fcn : DiscreteTransferFcn  Numerator=cell2mat(Peaking_inv_d(1,1).Num)  Denominator=cell2mat(Peaking_inv_d(1,1).Den)
  Discrete Transfer Fcn1 : DiscreteTransferFcn  Numerator=cell2mat(Peaking_inv_d(1,2).Num)  Denominator=cell2mat(Peaking_inv_d(1,2).Den)
  Discrete Transfer Fcn2 : DiscreteTransferFcn  Numerator=cell2mat(Peaking_inv_d(2,1).Num)  Denominator=cell2mat(Peaking_inv_d(2,1).Den)
  Discrete Transfer Fcn3 : DiscreteTransferFcn  Numerator=cell2mat(Peaking_inv_d(2,2).Num)  Denominator=cell2mat(Peaking_inv_d(2,2).Den)
  Mux1 : Mux  Inputs=2
  Scope : Subsystem  LoadFcn=plecs('sl', 300);  InitFcn=plecs('sl', 314);  StartFcn=plecs('sl', 308);  StopFcn=plecs('sl', 309);  mask{Settings=<binary blob, 216 chars, not shown>}
      mask init:
      | plecs('sl', 315);
      settings: CopyFcn=plecs('sl', 303);  DeleteFcn=plecs('sl', 305);  UndoDeleteFcn=plecs('sl', 306);  PreSaveFcn=plecs('sl', 311);  NameChangeFcn=plecs('sl', 310);  DestroyFcn=plecs('sl', 307);  OpenFcn=plecs('sl', 302);  ErrorFcn=plerrorfcn
      mask Display: plot([0.1 0.9 0.9 0.1 0.1], [0.9 0.9 0.5 0.5 0.9])
  Sum3 : Sum  Inputs=|++
  Sum4 : Sum  Inputs=|++
  Out1 : Outport
  wires:
  Demux/1 -> Discrete Transfer Fcn2/1, Discrete Transfer Fcn/1
  Demux/2 -> Discrete Transfer Fcn1/1, Discrete Transfer Fcn3/1
  Discrete Transfer Fcn2/1 -> Sum4/1
  Sum4/1 -> Mux1/2
  Mux1/1 -> Out1/1
  Sum3/1 -> Mux1/1, Scope/1(1)
  Discrete Transfer Fcn/1 -> Sum3/1
  Discrete Transfer Fcn1/1 -> Sum3/2
  In2/1 -> Demux/1
  Discrete Transfer Fcn3/1 -> Sum4/2

== system Filter_attivo/Controllo tensione/Controllo PR 10 kHz/Controllo risonante/Inversa ==
  1 : Inport
  2 : Inport  Port=2
  " 1 " : DataTypeConversion  SaturateOnIntegerOverflow=on  RndMeth=Zero
  " 2 " : DataTypeConversion  SaturateOnIntegerOverflow=on  RndMeth=Zero
  " InputMux " : Mux  Inputs=2
  " S-Function " : S-Function  FunctionName=plecs  SFunctionDeploymentMode=off  EnableBusSupport=off
  wires:
  " InputMux "/1 -> " S-Function "/1
  1/1 -> " 1 "/1
  " 1 "/1 -> " InputMux "/1
  2/1 -> " 2 "/1
  " 2 "/1 -> " InputMux "/2

== system Filter_attivo/Controllo tensione/Controllo PR 10 kHz/Controllo risonante/T_inversa ==
  dq : Inport
  teta : Inport  Port=2
  Demux : Demux  Outputs=2
  Fcn : Fcn  Expr=cos(u[3])*u[1]+sin(u[3])*u[2]
  Fcn1 : Fcn  Expr=-sin(u[3])*u[1]+cos(u[3])*u[2]
  Gain8 : Gain  Gain=-1
  Mux : Mux  Inputs=3
  Mux1 : Mux  Inputs=2
  dq(0) : Outport
  wires:
  dq/1 -> Demux/1
  Demux/1 -> Mux/1
  Demux/2 -> Mux/2
  Mux/1 -> Fcn/1, Fcn1/1
  Fcn/1 -> Mux1/1
  Fcn1/1 -> Mux1/2
  Mux1/1 -> dq(0)/1
  teta/1 -> Gain8/1
  Gain8/1 -> Mux/3

== system Filter_attivo/Controllo tensione/Controllo PR 10 kHz/PLL_tempo_discreto/D ==
  ab(c) : Inport
  Gain : Gain  Gain=[1 0; 1/sqrt(3) 2/sqrt(3)]  Multiplication=Matrix(K*u)
  dq(0) : Outport
  wires:
  Gain/1 -> dq(0)/1
  ab(c)/1 -> Gain/1

== system Filter_attivo/Controllo tensione/Controllo PR 10 kHz/PLL_tempo_discreto/Integratore discreto con reset a 2*pi ==
  omega : Inport
  Add : Sum
  Compare To Zero : simulink/Logic and Bit Operations/Compare To Zero  relop=>  OutDataTypeStr=uint8  ZeroCross=off
  Constant : Constant  Value=2*pi
  Constant1 : Constant  Value=-2*pi
  Constant2 : Constant  Value=-2*pi
  Constant3 : Constant  Value=2*pi
  Discrete-Time Integrator : DiscreteIntegrator  ExternalReset=rising  InitialConditionSource=external  SampleTime=-1  ShowStatePort=on  ICPrevOutput=DiscIntNeverNeededParam  ICPrevScaledInput=DiscIntNeverNeededParam
  Logical Operator2 : Logic  Operator=OR  AllPortsSameDT=off  OutDataTypeStr=boolean
  Relational Operator : RelationalOperator  Operator=<=  OutDataTypeStr=boolean  RndMeth=Nearest
  Relational Operator1 : RelationalOperator  Operator=<=  OutDataTypeStr=boolean  RndMeth=Nearest
  Switch : Switch  Threshold=0.5
  teta : Outport
  wires:
  Logical Operator2/1 -> Discrete-Time Integrator/2
  Relational Operator/1 -> Logical Operator2/1
  Relational Operator1/1 -> Logical Operator2/2
  Discrete-Time Integrator/State -> Add/1, Compare To Zero/1, Relational Operator1/1, Relational Operator/2
  Constant/1 -> Relational Operator/1
  Constant1/1 -> Relational Operator1/2
  omega/1 -> Discrete-Time Integrator/1
  Discrete-Time Integrator/1 -> teta/1
  Constant2/1 -> Switch/1
  Constant3/1 -> Switch/3
  Switch/1 -> Add/2
  Compare To Zero/1 -> Switch/2
  Add/1 -> Discrete-Time Integrator/3

== system Filter_attivo/Controllo tensione/Controllo PR 10 kHz/PLL_tempo_discreto/PI antiwindup ==
  In : Inport
  Constant : Constant  Value=kp_PLL_edit
  Constant1 : Constant  Value=ki_PLL_edit
  Constant2 : Constant  Value=min_PLL
  Constant3 : Constant  Value=max_PLL
  Constant4 : Constant  Value=kp_PLL
  Constant5 : Constant  Value=ki_PLL
  Embedded MATLAB Function : MATLAB Function  TreatAsAtomicUnit=on
  Out : Outport
  wires:
  Embedded MATLAB Function/1(out) -> Out/1
  Constant3/1 -> Embedded MATLAB Function/5(max)
  Constant2/1 -> Embedded MATLAB Function/4(min)
  Constant1/1 -> Embedded MATLAB Function/3(ki)
  Constant/1 -> Embedded MATLAB Function/2(kp)
  In/1 -> Embedded MATLAB Function/1(error)

== system Filter_attivo/Controllo tensione/Controllo PR 10 kHz/PLL_tempo_discreto/Scope ==
  1 : Inport
  2 : Inport  Port=2
  " 1 " : DataTypeConversion  SaturateOnIntegerOverflow=on  RndMeth=Zero
  " 2 " : DataTypeConversion  SaturateOnIntegerOverflow=on  RndMeth=Zero
  " InputMux " : Mux  Inputs=2
  " S-Function " : S-Function  FunctionName=plecs  SFunctionDeploymentMode=off  EnableBusSupport=off
  wires:
  " InputMux "/1 -> " S-Function "/1
  1/1 -> " 1 "/1
  " 1 "/1 -> " InputMux "/1
  2/1 -> " 2 "/1
  " 2 "/1 -> " InputMux "/2

== system Filter_attivo/Controllo tensione/Controllo PR 10 kHz/PLL_tempo_discreto/Subsystem ==
  vr : Inport
  FILTRO peaking diretta_prima : Subsystem
  notch_prima_tensione : Subsystem
  vr_prima(0) : Outport
  vr_armoniche(0) : Outport  Port=2
  wires:
  FILTRO peaking diretta_prima/1(Out1) -> vr_prima(0)/1
  vr/1 -> notch_prima_tensione/1(In1), FILTRO peaking diretta_prima/1(In2)
  notch_prima_tensione/1(Out1) -> vr_armoniche(0)/1

== system Filter_attivo/Controllo tensione/Controllo PR 10 kHz/PLL_tempo_discreto/T ==
  dq : Inport
  teta : Inport  Port=2
  Demux : Demux  Outputs=2
  Fcn : Fcn  Expr=cos(u[3])*u[1]+sin(u[3])*u[2]
  Fcn1 : Fcn  Expr=-sin(u[3])*u[1]+cos(u[3])*u[2]
  Mux : Mux  Inputs=3
  Mux1 : Mux  Inputs=2
  dq(teta) : Outport
  wires:
  Mux1/1 -> dq(teta)/1
  Fcn1/1 -> Mux1/2
  Fcn/1 -> Mux1/1
  Mux/1 -> Fcn/1, Fcn1/1
  teta/1 -> Mux/3
  Demux/2 -> Mux/2
  Demux/1 -> Mux/1
  dq/1 -> Demux/1

== system Filter_attivo/Controllo tensione/Controllo PR 10 kHz/PLL_tempo_discreto/Teta ==
  1 : Inport
  2 : Inport  Port=2
  " 1 " : DataTypeConversion  SaturateOnIntegerOverflow=on  RndMeth=Zero
  " 2 " : DataTypeConversion  SaturateOnIntegerOverflow=on  RndMeth=Zero
  " InputMux " : Mux  Inputs=2
  " S-Function " : S-Function  FunctionName=plecs  SFunctionDeploymentMode=off  EnableBusSupport=off
  wires:
  " InputMux "/1 -> " S-Function "/1
  1/1 -> " 1 "/1
  " 1 "/1 -> " InputMux "/1
  2/1 -> " 2 "/1
  " 2 "/1 -> " InputMux "/2

== system Filter_attivo/Controllo tensione/Controllo PR 10 kHz/PLL_tempo_discreto/vd_vq ==
  1 : Inport
  2 : Inport  Port=2
  " 1 " : DataTypeConversion  SaturateOnIntegerOverflow=on  RndMeth=Zero
  " 2 " : DataTypeConversion  SaturateOnIntegerOverflow=on  RndMeth=Zero
  " InputMux " : Mux  Inputs=2
  " S-Function " : S-Function  FunctionName=plecs  SFunctionDeploymentMode=off  EnableBusSupport=off
  wires:
  " 2 "/1 -> " InputMux "/2
  2/1 -> " 2 "/1
  " 1 "/1 -> " InputMux "/1
  1/1 -> " 1 "/1
  " InputMux "/1 -> " S-Function "/1

== system Filter_attivo/Controllo tensione/Controllo PR 10 kHz/Scope/ InputMux  ==
  In1 : Inport
  Convert1 : DataTypeConversion  SaturateOnIntegerOverflow=on  RndMeth=Zero
  Mux : Mux  Inputs=1
  Out : Outport
  wires:
  Convert1/1 -> Mux/1
  In1/1 -> Convert1/1
  Mux/1 -> Out/1

== system Filter_attivo/Controllo tensione/Controllo PR 10 kHz/controllo /PI antiwindup ==
  In : Inport
  Constant : Constant  Value=kp_rifasamento
  Constant1 : Constant  Value=ki_rifasamento
  Constant2 : Constant  Value=-10
  Constant3 : Constant  Value=10
  Embedded MATLAB Function : MATLAB Function  TreatAsAtomicUnit=on
  Out : Outport
  wires:
  In/1 -> Embedded MATLAB Function/1(error)
  Constant/1 -> Embedded MATLAB Function/2(kp)
  Constant1/1 -> Embedded MATLAB Function/3(ki)
  Constant2/1 -> Embedded MATLAB Function/4(min)
  Constant3/1 -> Embedded MATLAB Function/5(max)
  Embedded MATLAB Function/1(out) -> Out/1

== system Filter_attivo/Controllo tensione/Controllo PR 10 kHz/controllo /Scope ==
  1 : Inport
  " InputMux " : Subsystem
      mask Display: disp('Mux')
  " S-Function " : S-Function  FunctionName=plecs  SFunctionDeploymentMode=off  EnableBusSupport=off
  wires:
  1/1 -> " InputMux "/1(In1)
  " InputMux "/1(Out) -> " S-Function "/1

== system Filter_attivo/Controllo tensione/Controllo PR 10 kHz/controllo /Scope1 ==
  1 : Inport
  " InputMux " : Subsystem
      mask Display: disp('Mux')
  " S-Function " : S-Function  FunctionName=plecs  SFunctionDeploymentMode=off  EnableBusSupport=off
  wires:
  " InputMux "/1(Out) -> " S-Function "/1
  1/1 -> " InputMux "/1(In1)

== system Filter_attivo/Controllo tensione/Controllo PR 10 kHz/controllo /Scope2 ==
  1 : Inport
  " InputMux " : Subsystem
      mask Display: disp('Mux')
  " S-Function " : S-Function  FunctionName=plecs  SFunctionDeploymentMode=off  EnableBusSupport=off
  wires:
  1/1 -> " InputMux "/1(In1)
  " InputMux "/1(Out) -> " S-Function "/1

== system Filter_attivo/Controllo tensione/Controllo PR 10 kHz/controllo /Scope3 ==
  1 : Inport
  " InputMux " : Subsystem
      mask Display: disp('Mux')
  " S-Function " : S-Function  FunctionName=plecs  SFunctionDeploymentMode=off  EnableBusSupport=off
  wires:
  " InputMux "/1(Out) -> " S-Function "/1
  1/1 -> " InputMux "/1(In1)

== system Filter_attivo/Controllo tensione/Controllo PR 10 kHz/controllo /T ==
  dq : Inport
  teta : Inport  Port=2
  Demux : Demux  Outputs=2
  Fcn : Fcn  Expr=cos(u[3])*u[1]+sin(u[3])*u[2]
  Fcn1 : Fcn  Expr=-sin(u[3])*u[1]+cos(u[3])*u[2]
  Mux : Mux  Inputs=3
  Mux1 : Mux  Inputs=2
  dq(teta) : Outport
  wires:
  Mux1/1 -> dq(teta)/1
  Fcn1/1 -> Mux1/2
  Fcn/1 -> Mux1/1
  Mux/1 -> Fcn/1, Fcn1/1
  teta/1 -> Mux/3
  Demux/2 -> Mux/2
  Demux/1 -> Mux/1
  dq/1 -> Demux/1

== system Filter_attivo/Controllo tensione/Controllo PR 10 kHz/controllo bus DC/Filtro passa-basso tempo discreto ==
  In : Inport
  Avvio Inverter : Inport  Port=2
  "Vdc " : Inport  Port=3
  Constant : Constant  Value=tau_filtro_Vdc_ref
  Embedded MATLAB Function : MATLAB Function  TreatAsAtomicUnit=on
  Vdc*_filtrata : Outport
  wires:
  In/1 -> Embedded MATLAB Function/1(in)
  Embedded MATLAB Function/1(out) -> Vdc*_filtrata/1
  Constant/1 -> Embedded MATLAB Function/2(tau)
  "Vdc "/1 -> Embedded MATLAB Function/3(Vdc)
  Avvio Inverter/1 -> Embedded MATLAB Function/4(avvio)

== system Filter_attivo/Controllo tensione/Controllo PR 10 kHz/controllo bus DC/PI antiwindup ==
  In : Inport
  Constant : Constant  Value=kp_PI
  Constant1 : Constant  Value=ki_PI
  Constant2 : Constant  Value=min_PI
  Constant3 : Constant  Value=max_PI
  Embedded MATLAB Function : MATLAB Function  TreatAsAtomicUnit=on
  Out : Outport
  wires:
  Embedded MATLAB Function/1(out) -> Out/1
  Constant3/1 -> Embedded MATLAB Function/5(max)
  Constant2/1 -> Embedded MATLAB Function/4(min)
  Constant1/1 -> Embedded MATLAB Function/3(ki)
  Constant/1 -> Embedded MATLAB Function/2(kp)
  In/1 -> Embedded MATLAB Function/1(error)

== system Filter_attivo/Controllo tensione/Controllo PR 10 kHz/controllo bus DC/PI antiwindup1 ==
  In : Inport
  Constant : Constant  Value=kp_rifasamento
  Constant1 : Constant  Value=ki_rifasamento
  Constant4 : Constant  Value=min_PI
  Constant5 : Constant  Value=max_PI
  Embedded MATLAB Function : MATLAB Function  TreatAsAtomicUnit=on
  Out : Outport
  wires:
  In/1 -> Embedded MATLAB Function/1(error)
  Constant/1 -> Embedded MATLAB Function/2(kp)
  Constant1/1 -> Embedded MATLAB Function/3(ki)
  Embedded MATLAB Function/1(out) -> Out/1
  Constant4/1 -> Embedded MATLAB Function/4(min)
  Constant5/1 -> Embedded MATLAB Function/5(max)

== system Filter_attivo/Controllo tensione/Controllo PR 10 kHz/controllo bus DC/Scope1 ==
  1 : Inport
  " 1 " : DataTypeConversion  SaturateOnIntegerOverflow=on  RndMeth=Zero
  " InputMux " : Mux  Inputs=1
  " S-Function " : S-Function  FunctionName=plecs  SFunctionDeploymentMode=off  EnableBusSupport=off
  wires:
  " InputMux "/1 -> " S-Function "/1
  1/1 -> " 1 "/1
  " 1 "/1 -> " InputMux "/1

== system Filter_attivo/Controllo tensione/Controllo PR 10 kHz/controllo bus DC/Scope2 ==
  1 : Inport
  2 : Inport  Port=2
  " 1 " : DataTypeConversion  SaturateOnIntegerOverflow=on  RndMeth=Zero
  " 2 " : DataTypeConversion  SaturateOnIntegerOverflow=on  RndMeth=Zero
  " InputMux " : Mux  Inputs=2
  " S-Function " : S-Function  FunctionName=plecs  SFunctionDeploymentMode=off  EnableBusSupport=off
  wires:
  " InputMux "/1 -> " S-Function "/1
  1/1 -> " 1 "/1
  " 1 "/1 -> " InputMux "/1
  2/1 -> " 2 "/1
  " 2 "/1 -> " InputMux "/2

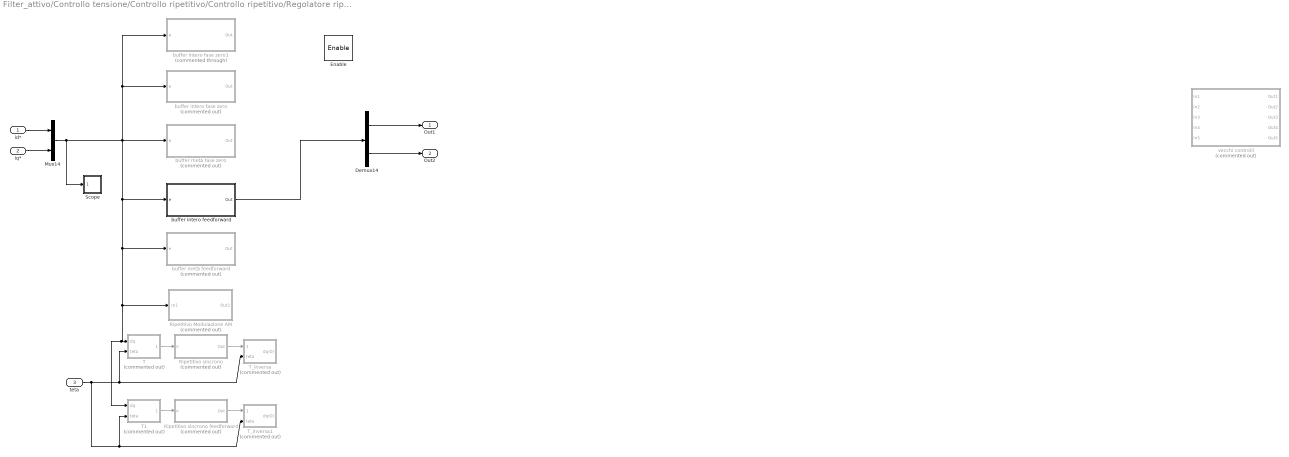
== system Filter_attivo/Controllo tensione/Controllo ripetitivo/Controllo ripetitivo/Regolatore ripetitivo ==
  id* : Inport
  iq* : Inport  Port=2
  teta : Inport  Port=3
  Enable : EnablePort  StatesWhenEnabling=reset
  " Ripetitivo sincrono" : Subsystem  Commented=on  mask{ro=4, rit=4, k_ser_=15}
      mask prompts: ro "Riduzione Buffer"; rit "Cicli compensati inverter"; k_ser_ "k serie"
  " Ripetitivo sincrono feedforward" : Subsystem  Commented=on  mask{ro=4, rit=4, k_ser_=5}
      mask prompts: ro "Riduzione Buffer"; rit "Cicli compensati inverter"; k_ser_ "k serie"
  " buffer intero fase zero" : Subsystem  Commented=on  mask{ro=1, rit=4, k_serie=5}
      mask prompts: ro "Riduzione Buffer"; rit "cicli compensati"
  " buffer intero fase zero1" : Subsystem  Commented=through  mask{ro=1, rit=1, k_serie=5}
      mask prompts: ro "Riduzione Buffer"; rit "cicli compensati"
  " buffer intero feedforward" : Subsystem  mask{ro=1, rit=2, k_serie=2}
      mask prompts: ro "Riduzione Buffer"; rit "cicli compensati"
  " buffer metà fase zero" : Subsystem  Commented=on  mask{ro=2, rit=4, k_serie=5}
      mask prompts: ro "Riduzione Buffer"; rit "cicli compensati"
  " buffer metà feedforward" : Subsystem  Commented=on  mask{ro=2, rit=2, k_serie=2}
      mask prompts: ro "Riduzione Buffer"; rit "cicli compensati"
  Demux14 : Demux  Outputs=2
  Mux14 : Mux  Inputs=2
  Ripetitivo Modulazione AM : Subsystem  Commented=on
  Scope : Subsystem  LoadFcn=plecs('sl', 300);  InitFcn=plecs('sl', 314);  StartFcn=plecs('sl', 308);  StopFcn=plecs('sl', 309);  mask{Settings=<binary blob, 892 chars, not shown>}
      mask init:
      | plecs('sl', 315);
      settings: CopyFcn=plecs('sl', 303);  DeleteFcn=plecs('sl', 305);  UndoDeleteFcn=plecs('sl', 306);  PreSaveFcn=plecs('sl', 311);  NameChangeFcn=plecs('sl', 310);  DestroyFcn=plecs('sl', 307);  OpenFcn=plecs('sl', 302);  ErrorFcn=plerrorfcn
      mask Display: plot([0.1 0.9 0.9 0.1 0.1], [0.9 0.9 0.5 0.5 0.9])
  T : Subsystem  Commented=on
  T1 : Subsystem  Commented=on
  T_inversa : Subsystem  Commented=on
  T_inversa1 : Subsystem  Commented=on
  vecchi controlli : Subsystem  Commented=on
  Out1 : Outport
  Out2 : Outport  Port=2
  wires:
  id*/1 -> Mux14/1
  iq*/1 -> Mux14/2
  Demux14/1 -> Out1/1
  Demux14/2 -> Out2/1
  T/1(dq(teta)) -> " Ripetitivo sincrono"/1(ir)
  " Ripetitivo sincrono"/1(Out) -> T_inversa/1(dq(teta))
  T1/1(dq(teta)) -> " Ripetitivo sincrono feedforward"/1(ir)
  " Ripetitivo sincrono feedforward"/1(Out) -> T_inversa1/1(dq(teta))
  teta/1 -> T1/2(teta), T_inversa1/2(teta), T/2(teta), T_inversa/2(teta)
  Mux14/1 -> Scope/1(1), " buffer intero fase zero1"/1(e), " buffer intero fase zero"/1(e), " buffer metà fase zero"/1(e), Ripetitivo Modulazione AM/1(In1), T1/1(dq), T/1(dq), " buffer metà feedforward"/1(e), " buffer intero feedforward"/1(e)
  " buffer intero feedforward"/1(Out) -> Demux14/1

== system Filter_attivo/Controllo tensione/Controllo ripetitivo/Controllo ripetitivo con downsampling/Regolatore ripetitivo ==
  note: Buffer Intero-feedforward
  note: Buffer Intero
  note: Buffer metà
  id* : Inport
  iq* : Inport  Port=2
  Enable : EnablePort  StatesWhenEnabling=reset
  " buffer intero fase zero" : Subsystem  mask{ro=down, rit=2, k_serie=k_serie_d}
      mask prompts: ro "Riduzione Buffer"; rit "cicli compensati"
  " buffer intero fase zero-riduzione di 1" : Subsystem  mask{ro=down, rit=2, k_serie=k_serie_d}
      mask prompts: ro "Riduzione Buffer"; rit "cicli compensati"
  " buffer intero fase zero-riduzione di 3" : Subsystem  mask{ro=down, rit=2, k_serie=k_serie_d}
      mask prompts: ro "Riduzione Buffer"; rit "cicli compensati"
  " buffer intero mattavelli" : Subsystem  mask{ro=down, rit=2, k_serie=5}
      mask prompts: ro "Riduzione Buffer"; rit "cicli compensati"
  " buffer intero mattavelli-riduzione di 3" : Subsystem  mask{ro=down, rit=2, k_serie=5}
      mask prompts: ro "Riduzione Buffer"; rit "cicli compensati"
  " buffer metà fase zero" : Subsystem  mask{ro=2, rit=2, k_serie=k_serie_d}
      mask prompts: ro "Riduzione Buffer"; rit "cicli compensati"
  " buffer metà fase zero-riduzione di 3" : Subsystem  mask{ro=2, rit=2, k_serie=k_serie_d}
      mask prompts: ro "Riduzione Buffer"; rit "cicli compensati"
  " buffer metà mattavelli" : Subsystem  mask{ro=2, rit=2, k_serie=5}
      mask prompts: ro "Riduzione Buffer"; rit "cicli compensati"
  Demux14 : Demux  Outputs=2
  Mux14 : Mux  Inputs=2
  Scope : Subsystem  LoadFcn=plecs('sl', 300);  InitFcn=plecs('sl', 314);  StartFcn=plecs('sl', 308);  StopFcn=plecs('sl', 309);  mask{Settings=<binary blob, 216 chars, not shown>}
      mask init:
      | plecs('sl', 315);
      settings: CopyFcn=plecs('sl', 303);  DeleteFcn=plecs('sl', 305);  UndoDeleteFcn=plecs('sl', 306);  PreSaveFcn=plecs('sl', 311);  NameChangeFcn=plecs('sl', 310);  DestroyFcn=plecs('sl', 307);  OpenFcn=plecs('sl', 302);  ErrorFcn=plerrorfcn
      mask Display: plot([0.1 0.9 0.9 0.1 0.1], [0.9 0.9 0.5 0.5 0.9])
  Out1 : Outport
  Out2 : Outport  Port=2
  wires:
  id*/1 -> Mux14/1
  iq*/1 -> Mux14/2
  Demux14/1 -> Out1/1
  Demux14/2 -> Out2/1
  Mux14/1 -> Scope/1(1), " buffer intero fase zero-riduzione di 3"/1(ir_h), " buffer intero fase zero"/1(e), " buffer intero mattavelli-riduzione di 3"/1(e), " buffer metà mattavelli"/1(e), " buffer intero mattavelli"/1(e), " buffer metà fase zero"/1(e), " buffer metà fase zero-riduzione di 3"/1(e)
  " buffer intero fase zero-riduzione di 3"/1(Out) -> Demux14/1
